simulink model "untitled"  (R2016a)
settings: Solver=VariableStepAuto  StartTime=0.0  StopTime=10.0  RelTol=1e-3
settings Model: Creator=ABHISHEK GOEL  LastModifiedBy=ABHISHEK GOEL

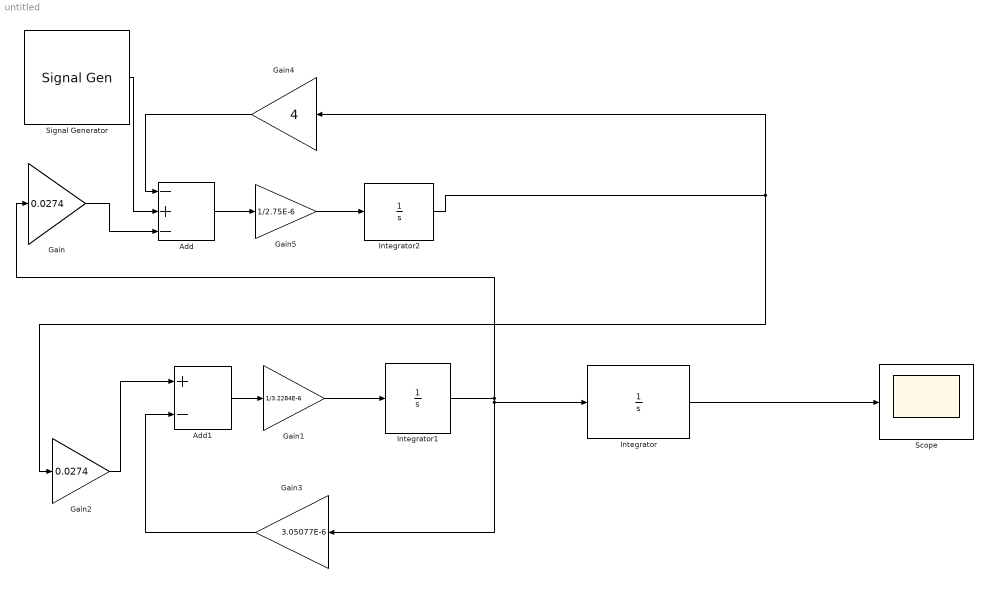
== system untitled ==
  Add : Sum  Inputs=-+-
  Add1 : Sum  Inputs=+-
  Gain : Gain  Gain=0.0274
  Gain1 : Gain  Gain=1/3.2284E-6
  Gain2 : Gain  Gain=0.0274
  Gain3 : Gain  Gain=3.05077E-6
  Gain4 : Gain  Gain=4
  Gain5 : Gain  Gain=1/2.75E-6
  Integrator : Integrator
  Integrator1 : Integrator
  Integrator2 : Integrator
  Scope : Scope
  Signal Generator : SignalGenerator  Amplitude=10  Frequency=10
  wires:
  Gain/1 -> Add/3
  Signal Generator/1 -> Add/2
  Gain4/1 -> Add/1
  Add/1 -> Gain5/1
  Gain5/1 -> Integrator2/1
  Integrator/1 -> Scope/1
  Integrator1/1 -> Gain3/1, Integrator/1, Gain/1
  Gain1/1 -> Integrator1/1
  Add1/1 -> Gain1/1
  Gain2/1 -> Add1/1
  Gain3/1 -> Add1/2
  Integrator2/1 -> Gain2/1, Gain4/1
